simulink model "Statedrivestepper"  (R2020a)
settings: Solver=FixedStepAuto  StartTime=0.0  StopTime=inf  RelTol=1e-3  EnableMultiTasking=on
libraries: mbedblockslib x10
settings Model: SILPILModeSetting=veronly  ExtModeTrigDuration=10  Creator=matas  LastModifiedBy=matas
settings OptimizationCC: EnhancedBackFolding=on  PassReuseOutputArgsAs=Individual arguments  ZeroExternalMemoryAtStartup=off  ZeroInternalMemoryAtStartup=off  MaxStackSize=64  OptimizeBlockOrder=speed  DifferentSizesBufferReuse=on  OptimizationCustomize=off  EfficientTunableParamExpr=on
settings DebuggingCC: ParameterTunabilityLossMsg=error
settings HardwareCC: ProdBitPerPointer=32  ProdBitPerSizeT=32  ProdBitPerPtrDiffT=32  ProdLargestAtomicInteger=Long  ProdLargestAtomicFloat=Double  ProdWordSize=32  ProdHWDeviceType=ARM Compatible->ARM Cortex
settings SFSimCC: MATLABDynamicMemAlloc=off
settings RTWCC: SystemTargetFile=ert.tlc  HardwareBoard=STM32 Nucleo F411RE  TLCOptions=-aInlineSetEventsForThisBaseRateFcn=TLC_FALSE -aSuppressMultiTaskScheduler=TLC_FALSE -aRateBasedStepFcn=1  TemplateMakefile=ert_default_tmf  Toolchain=GNU Tools for ARM Embedded Processors
settings CodeAppCC: ForceParamTrailComments=on  IgnoreCustomStorageClasses=off  OperatorAnnotations=on  SimulinkDataObjDesc=on  SFDataObjDesc=on  InsertBlockDesc=on
settings ERTTargetCC: SupportContinuousTime=on  ExtModeStaticAllocSize=2000

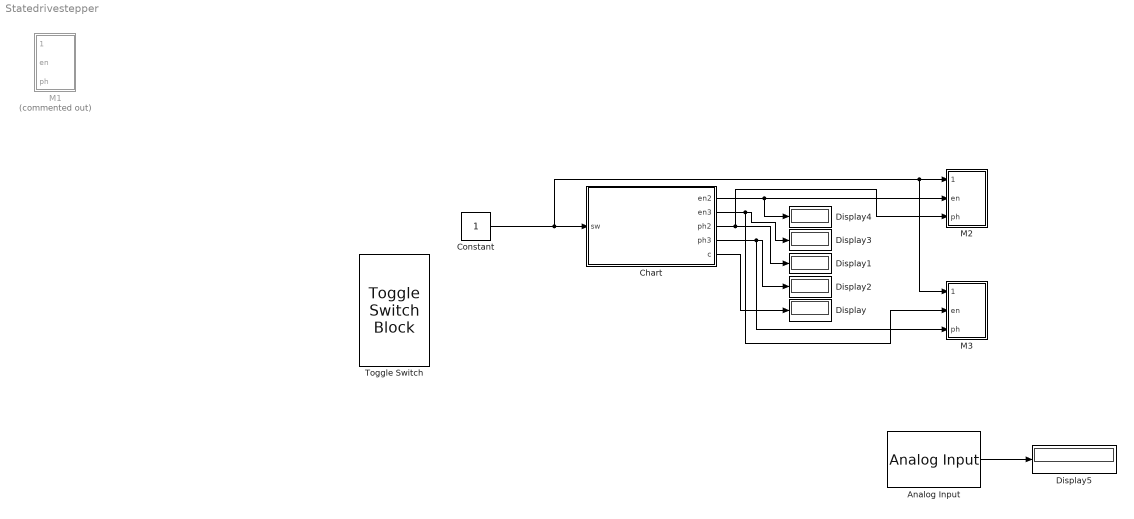
== system Statedrivestepper ==
  Analog Input : mbedblockslib/Analog Input  Pin=PA_7  ReadResultsOnly=off  ConversionTriggerSource=Software  ExternalTriggerType=uint32( 0 )  OutputDataType=double  EnableConversionCompleteNotify=off  EnableOuputStatus=off  SampleTime=-1
      settings: SourceProductBaseCode=MICROBIT,NUCLEO,STMICRODIS
  Chart : Stateflow chart  TreatAsAtomicUnit=on
  Constant : Constant
  Display{,1..5} (6 alike) : Display
  M1 : Subsystem  Commented=on
  M2 : Subsystem
  M3 : Subsystem
  Toggle Switch : ToggleSwitchBlock
      settings: Values={{'Off', 'On'}, [0 1]}
  wires:
  Constant/1 -> M3/1(nsleep), M2/1(nsleep), Chart/1(sw)
  Chart/5(c) -> Display/1
  Chart/4(ph3) -> M3/3(ph), Display2/1
  Chart/3(ph2) -> M2/3(ph), Display1/1
  Chart/2(en3) -> M3/2(en), Display3/1
  Chart/1(en2) -> M2/2(en), Display4/1
  Analog Input/1 -> Display5/1

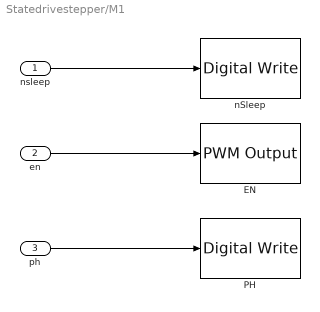
== system Statedrivestepper/M1 ==
  nsleep : Inport
  en : Inport  Port=2
  ph : Inport  Port=3
  EN : mbedblockslib/PWM Output  Pin=PC_8  EnableInputFrequency=off  InitialFrequency=500  InitialDutyCycle=50  NotificationType=None
      settings: SourceProductBaseCode=MICROBIT,NUCLEO,STMICRODIS
  PH : mbedblockslib/Digital Write  Pin=PC_6  Direction=output
      settings: SourceProductBaseCode=MICROBIT,NUCLEO,STMICRODIS
  nSleep : mbedblockslib/Digital Write  Pin=PA_12  Direction=output
      settings: SourceProductBaseCode=MICROBIT,NUCLEO,STMICRODIS
  wires:
  ph/1 -> PH/1
  en/1 -> EN/1
  nsleep/1 -> nSleep/1

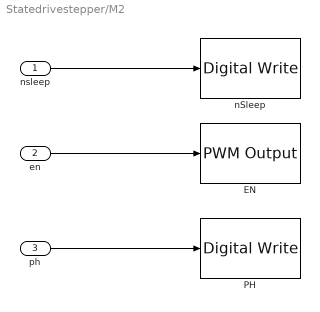
== system Statedrivestepper/M2 ==
  nsleep : Inport
  en : Inport  Port=2
  ph : Inport  Port=3
  EN : mbedblockslib/PWM Output  Pin=PA_11  EnableInputFrequency=off  InitialFrequency=500  InitialDutyCycle=50  NotificationType=None
      settings: SourceProductBaseCode=MICROBIT,NUCLEO,STMICRODIS
  PH : mbedblockslib/Digital Write  Pin=PC_7  Direction=output
      settings: SourceProductBaseCode=MICROBIT,NUCLEO,STMICRODIS
  nSleep : mbedblockslib/Digital Write  Pin=PB_2  Direction=output
      settings: SourceProductBaseCode=MICROBIT,NUCLEO,STMICRODIS
  wires:
  ph/1 -> PH/1
  en/1 -> EN/1
  nsleep/1 -> nSleep/1

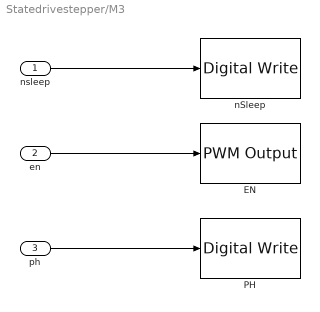
== system Statedrivestepper/M3 ==
  nsleep : Inport
  en : Inport  Port=2
  ph : Inport  Port=3
  EN : mbedblockslib/PWM Output  Pin=PA_9  EnableInputFrequency=off  InitialFrequency=500  InitialDutyCycle=50  NotificationType=None
      settings: SourceProductBaseCode=MICROBIT,NUCLEO,STMICRODIS
  PH : mbedblockslib/Digital Write  Pin=PB_10  Direction=output
      settings: SourceProductBaseCode=MICROBIT,NUCLEO,STMICRODIS
  nSleep : mbedblockslib/Digital Write  Pin=PB_15  Direction=output
      settings: SourceProductBaseCode=MICROBIT,NUCLEO,STMICRODIS
  wires:
  ph/1 -> PH/1
  en/1 -> EN/1
  nsleep/1 -> nSleep/1

== stateflow chart Statedrivestepper/Chart ==
  settings: updateMethod=DISCRETE  sampleTime=0.1
  state forward2
    during:
    c=c+1;
  state sleep
  state forward3
    during:
    c=c+1;
  forward2 -> forward3 [order 1] : [c==3]{ph2=1;
      | ph3=1;
      | en2=0;
      | en3=1;
      | c=0;}
  sleep -> forward2 : [sw==1]{ph2=1;
      | ph3=1;
      | en2=1;
      | en3=0;
      | c=0;}
  forward2 -> sleep [order 2] : [sw==0]{ph2=0;
      | ph3=0;
      | en2=0;
      | en3=0;
      | c=0;}
  forward3 -> forward2 : [c==3]{ph2=1;
      | ph3=1;
      | en2=1;
      | en3=0;
      | c=0;}
  (default) -> sleep : {en2=0;
      | en3=0;
      | ph2=0;
      | ph3=0;
      | c=0;}
  data: sw input; en2 output; en3 output; ph2 output; ph3 output; c output
